simulink model "Heating_System_control101"  (R2023a)
settings: Solver=ode45  StartTime=0.0  StopTime=10  RelTol=1e-3  EnableMultiTasking=on
settings Model: Creator=co1gp  LastModifiedBy=Anthony Rossiter
settings SolverCC: AlgebraicLoopSolver=TrustRegion
settings DataIOCC: LimitDataPoints=on  SaveFormat=Array  SignalLoggingSaveFormat=ModelDataLogs  ReturnWorkspaceOutputs=off
settings OptimizationCC: ExpressionDepthLimit=2147483647  LifeSpan=inf
settings DebuggingCC: UnderspecifiedInitializationDetection=Classic  MergeDetectMultiDrivingBlocksExec=none  SolverPrmCheckMsg=warning  FcnCallInpInsideContextMsg=warning  UnconnectedInputMsg=warning  UnconnectedOutputMsg=warning  UnconnectedLineMsg=warning  StateNameClashWarn=warning  SFUnexpectedBacktrackingDiag=warning  SFNoUnconditionalDefaultTransitionDiag=warning  SFExecutionAtInitializationDiag=none  ArithmeticOperatorsInVariantConditions=warning
settings HardwareCC: ProdBitPerPointer=32  ProdBitPerSizeT=32  ProdBitPerPtrDiffT=32  ProdLargestAtomicFloat=None  ProdIntDivRoundTo=Undefined  ProdEndianess=Unspecified  ProdWordSize=32  ProdHWDeviceType=32-bit Generic
settings ModelReferenceCC: EnableRefExpFcnMdlSchedulingChecks=on  PropagateSignalLabelsOutOfModel=off
settings SFSimCC: SimUseLocalCustomCode=off  CustomCodeUndefinedFunction=UseInterfaceOnly
settings RTWCC: RTWUseLocalCustomCode=off  DLArmComputeVersion=19.05
settings CodeAppCC: StateflowObjectComments=on
settings GRTTargetCC: TargetLangStandard=C89/C90 (ANSI)  CombineOutputUpdateFcns=off  GRTInterface=on
settings ConfigComp: CovMetricSettings=dw  CovSaveCumulativeToWorkspaceVar=on  CovSaveSingleToWorkspaceVar=on  CovExternalEMLEnable=off  CovSFcnEnable=off

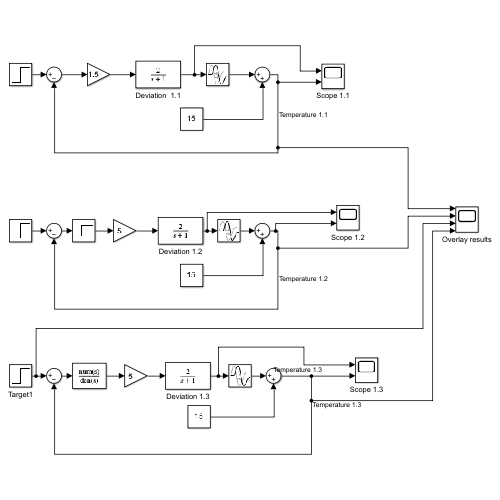
[thumbnail: Simulink's stored preview of the top-level diagram]
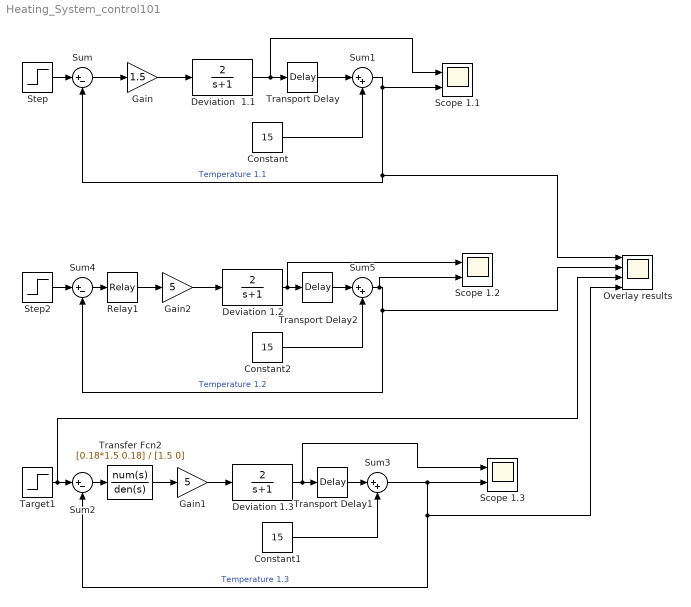
== system Heating_System_control101 ==
  Constant : Constant  Value=15
  Constant1 : Constant  Value=15
  Constant2 : Constant  Value=15
  Deviation  1.1 : TransferFcn  Numerator=[2]  Denominator=[1 1]
  Deviation 1.2 : TransferFcn  Numerator=[2]  Denominator=[1 1]
  Deviation 1.3 : TransferFcn  Numerator=[2]  Denominator=[1 1]
  Gain : Gain  Gain=1.5
  Gain1 : Gain  Gain=5
  Gain2 : Gain  Gain=5
  Overlay results : Scope  NumInputPorts=4
  Relay1 : Relay  OnSwitchValue=.1  OffSwitchValue=-.1
  Scope 1.1 : Scope  NumInputPorts=2
  Scope 1.2 : Scope  NumInputPorts=2
  Scope 1.3 : Scope  NumInputPorts=2
  Step : Step  Time=0.5  Before=15  After=20  SampleTime=0
  Step2 : Step  Time=0.5  Before=15  After=20  SampleTime=0
  Sum : Sum  Inputs=|+-
  Sum1 : Sum  Inputs=|++
  Sum2 : Sum  Inputs=|+-
  Sum3 : Sum  Inputs=|++
  Sum4 : Sum  Inputs=|+-
  Sum5 : Sum  Inputs=|++
  Target1 : Step  Time=0.5  Before=15  After=20  SampleTime=0
  Transfer Fcn2 : TransferFcn  Numerator=[0.18*1.5 0.18]  Denominator=[1.5 0]
  Transport Delay : TransportDelay  DelayTime=0.5
  Transport Delay1 : TransportDelay  DelayTime=0.5
  Transport Delay2 : TransportDelay  DelayTime=0.5
  wires:
  Sum/1 -> Gain/1
  Gain/1 -> Deviation  1.1/1
  Step/1 -> Sum/1
  Transport Delay/1 -> Sum1/1
  Constant/1 -> Sum1/2
  Sum1/1 -> Scope 1.1/2, Overlay results/1, Sum/2  "Temperature 1.1"
  Transfer Fcn2/1 -> Gain1/1
  Gain1/1 -> Deviation 1.3/1
  Target1/1 -> Overlay results/3, Sum2/1
  Sum2/1 -> Transfer Fcn2/1
  Deviation 1.3/1 -> Scope 1.3/1, Transport Delay1/1
  Transport Delay1/1 -> Sum3/1
  Constant1/1 -> Sum3/2
  Sum3/1 -> Sum2/2, Overlay results/4, Scope 1.3/2  "Temperature 1.3"
  Relay1/1 -> Gain2/1
  Gain2/1 -> Deviation 1.2/1
  Step2/1 -> Sum4/1
  Sum4/1 -> Relay1/1
  Deviation 1.2/1 -> Scope 1.2/1, Transport Delay2/1
  Transport Delay2/1 -> Sum5/1
  Constant2/1 -> Sum5/2
  Sum5/1 -> Scope 1.2/2, Sum4/2, Overlay results/2  "Temperature 1.2"
  Deviation  1.1/1 -> Scope 1.1/1, Transport Delay/1
